simulink model "test_CounterTrajIncrement"  (R2015b)
settings: Solver=FixedStepDiscrete  StartTime=0.0  StopTime=0.10  FixedStep=0.005  RelTol=1e-3
settings Model: Creator=jeljaik  LastModifiedBy=jeljaik

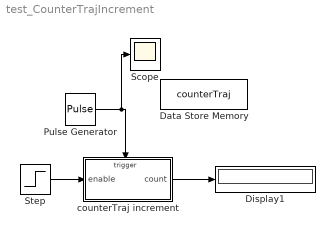
== system test_CounterTrajIncrement ==
  Data Store Memory : DataStoreMemory  Priority=1  DataStoreName=counterTraj  ReadBeforeWriteMsg=warning  WriteAfterWriteMsg=warning  WriteAfterReadMsg=warning  OutDataTypeStr=double
  Display1 : Display
  Pulse Generator : DiscretePulseGenerator  SampleTime=0.005
  Scope : Scope
  Step : Step  Time=0.05  SampleTime=0
  counterTraj increment : Subsystem  mask(counterTraj){}
      mask help:
      | Given a global variable 'counterTraj' defined through a 'Data Store Memory'
      | block, this block uses the 'Pulse Generator' to trigger the increment of
      | this variable if and only if the 'enable' signal is 1.
  wires:
  counterTraj increment/1(count) -> Display1/1
  Pulse Generator/1 -> Scope/1, counterTraj increment/Trigger
  Step/1 -> counterTraj increment/1(enable)

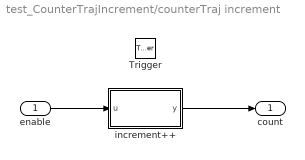
== system test_CounterTrajIncrement/counterTraj increment ==
  enable : Inport
  Trigger : TriggerPort  PortDimensions=1
  increment++ : MATLAB Function  TreatAsAtomicUnit=on
  count : Outport
  wires:
  enable/1 -> increment++/1(u)
  increment++/1(y) -> count/1

== matlab function test_CounterTrajIncrement/counterTraj increment/increment++ ==
  data: u input; y output; counterTraj data_store_memory
function y = fcn(u)
% If the input is 1 (if the corresponding state machine allows the
% increment of counterTraj, then it increments, otherwise, it remains the
% same. 
%#codegen
global counterTraj;

if u
    counterTraj = counterTraj + 1;
end

y = counterTraj;
